simulink model "BMS_BalancingLogic_COM"  (R2022b)
settings: configuration reference "BMS_Sw_CodeGenConfig" (kept outside this file)
model workspace: external: MAT-File H:\0\New MAAM\10 - MBD\Battary Management System\SWE.3 CDD\DataTypes\Data_Script.mat (data not in the file)
undefined symbols (not defined in the file): Schedule
settings Model: DataDictionary=BMS_Arch_DD.sldd  Creator=MAAM  LastModifiedBy=MAAM
settings ConfigSetRef: SourceName=BMS_Sw_CodeGenConfig

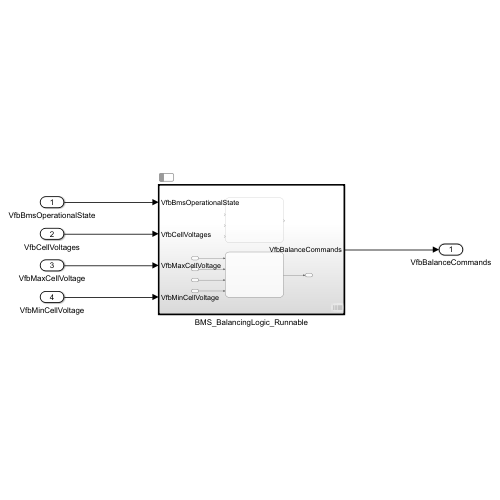
[thumbnail: Simulink's stored preview of the top-level diagram]
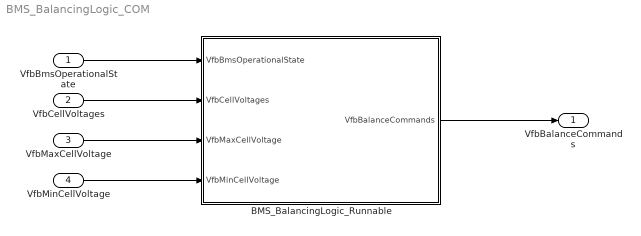
== system BMS_BalancingLogic_COM ==
  VfbBmsOperationalState : Inport
  VfbCellVoltages : Inport  Port=2
  VfbMaxCellVoltage : Inport  Port=3
  VfbMinCellVoltage : Inport  Port=4
  BMS_BalancingLogic_Runnable : Subsystem  Tag=BMS_BalancingLogic_Task  Priority=2  TreatAsAtomicUnit=on  ScheduleAs=Periodic partition  PartitionName=BMS_BalancingLogic_Task  SystemSampleTime=Schedule.BMS_BalancingLogic_Task
      settings: RTWSystemCode=Nonreusable function  RTWFcnNameOpts=Use subsystem name  RTWFileNameOpts=Use subsystem name  FunctionInterfaceSpec=Allow arguments (Optimized)
  VfbBalanceCommands : Outport
  wires:
  VfbBmsOperationalState/1 -> BMS_BalancingLogic_Runnable/1(VfbBmsOperationalState)
  VfbCellVoltages/1 -> BMS_BalancingLogic_Runnable/2(VfbCellVoltages)
  VfbMaxCellVoltage/1 -> BMS_BalancingLogic_Runnable/3(VfbMaxCellVoltage)
  VfbMinCellVoltage/1 -> BMS_BalancingLogic_Runnable/4(VfbMinCellVoltage)
  BMS_BalancingLogic_Runnable/1(VfbBalanceCommands) -> VfbBalanceCommands/1

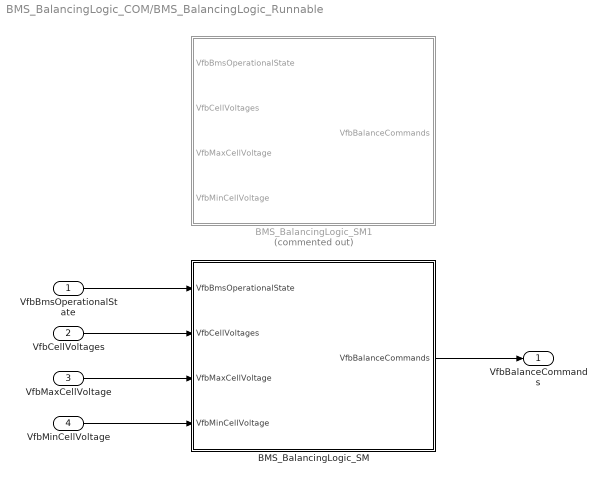
== system BMS_BalancingLogic_COM/BMS_BalancingLogic_Runnable ==
  VfbBmsOperationalState : Inport  OutDataTypeStr=Enum: BMS_State_Enum  PortDimensions=1
  VfbCellVoltages : Inport  Port=2
  VfbMaxCellVoltage : Inport  Port=3
  VfbMinCellVoltage : Inport  Port=4
  BMS_BalancingLogic_SM : Stateflow chart  TreatAsAtomicUnit=on
  BMS_BalancingLogic_SM1 : Stateflow chart  Commented=on  TreatAsAtomicUnit=on
  VfbBalanceCommands : Outport
  wires:
  VfbCellVoltages/1 -> BMS_BalancingLogic_SM/2(VfbCellVoltages)
  VfbMinCellVoltage/1 -> BMS_BalancingLogic_SM/4(VfbMinCellVoltage)
  BMS_BalancingLogic_SM/1(VfbBalanceCommands) -> VfbBalanceCommands/1
  VfbBmsOperationalState/1 -> BMS_BalancingLogic_SM/1(VfbBmsOperationalState)
  VfbMaxCellVoltage/1 -> BMS_BalancingLogic_SM/3(VfbMaxCellVoltage)

== stateflow chart BMS_BalancingLogic_COM/BMS_BalancingLogic_Runnable/BMS_BalancingLogic_SM ==
  state out  = ActivateBalancing(MAX, MIN, THR) [function]
    (default) -> (junction 25)
    (junction 25) -> (junction 26) [order 1] : [ (MAX - MIN) >= (THR - 1e-5) ]
    (junction 25) -> (junction 27) [order 2] : {out = false;}
    (junction 26) -> (junction 28) : {out = true;}
    (junction 28) -> (junction 27)
    (junction 27) -> (junction 29)
  state Balancing_Test [parallel]
    en, du:
    BalancingFlag = ActivateBalancing(VfbMaxCellVoltage, VfbMinCellVoltage, BalancingThreshold(state));
    settings: executionOrder=1
  state Balancing_Logic [parallel]
    settings: executionOrder=2
    state SW_Off
      en:
      VfbBalanceCommands(:,:) = false;
      state = 1;
    state Super
      state BalancingNotActive
        en:
        state = 1;
      state BalancingIsActive
        en, du:
        state = 2;
        VfbBalanceCommands(:,:) = boolean( (VfbCellVoltages - VfbMinCellVoltage)  > BalancingThreshold(state) );
        ex:
        VfbBalanceCommands(:,:) = false;
      (default) -> BalancingNotActive
      BalancingIsActive -> BalancingNotActive : [~BalancingFlag]
      BalancingNotActive -> BalancingIsActive [order 1] : [BalancingFlag]
    (default) -> SW_Off
    Super -> SW_Off : [VfbBmsOperationalState ~= BMS_State_Enum.BMS_Balancing]
    SW_Off -> Super : [BalancingFlag && ...
        | after(BalancingOffWait, sec)]
    BalancingNotActive -> SW_Off [order 2] : [after(BalancingOnWait, sec)]
  data: MAX function_input single size=1; out function_output boolean size=1; MIN function_input single size=1; THR function_input; VfbBmsOperationalState input Enum: BMS_State_Enum size=1; VfbCellVoltages input single size=BATT.Package.Ns_Module*BATT.Package.NumModules; VfbMaxCellVoltage input single size=1; VfbMinCellVoltage input single size=1; VfbBalanceCommands output boolean size=BATT.Package.Ns_Module*BATT.Package.NumModules =boolean(zeros(1,BATT.Package.Ns_Module*BATT.Package.NumModules))'; BalancingOffWait constant uint8 size=1 =BATT.Balancing.BalWaitOff; BalancingOnWait constant uint8 size=1 =BATT.Balancing.BalWaitOn; BalancingFlag local boolean size=1 =true; state local =1; BalancingThreshold constant single size=[1 2] =[BATT.Balancing.ThresholdOn , BATT.Balancing.ThresholdOff]

== stateflow chart BMS_BalancingLogic_COM/BMS_BalancingLogic_Runnable/BMS_BalancingLogic_SM1 ==
  state SW_Off
    en:
    VfbBalanceCommands(:,:) = false;
    du:
    BalancingFlag = ActivateBalancing(VfbMaxCellVoltage, VfbMinCellVoltage, BalancingThreshold_ON);
  state out  = ActivateBalancing(MAX, MIN, THR) [function]
    (default) -> (junction 25)
    (junction 25) -> (junction 26) [order 1] : [ (MAX - MIN) >= (THR - 1e-5) ]
    (junction 25) -> (junction 27) [order 2] : {out = false;}
    (junction 26) -> (junction 28) : {out = true;}
    (junction 28) -> (junction 27)
    (junction 27) -> (junction 29)
  state Super
    state BalancingNotActive
      en, du:
      BalancingFlag = ActivateBalancing(VfbMaxCellVoltage, VfbMinCellVoltage, BalancingThreshold_ON);
    state BalancingIsActive
      en, du:
      BalancingFlag = ActivateBalancing( ...
      VfbMaxCellVoltage, VfbMinCellVoltage, BalancingThreshold_OFF);
      ex:
      VfbBalanceCommands(:,:) = false;
      state BalancingActiveMode
        state SW1_On
          en:
          VfbBalanceCommands(1) = true;
          ex:
          VfbBalanceCommands(1) = false;
          step = 1;
        state SW_Wait
        state SW2_On
          en:
          VfbBalanceCommands(2) = true;
          ex:
          VfbBalanceCommands(2) = false;
          step = 2;
        (default) -> SW1_On
        SW_Wait -> SW1_On [order 1] : after((0.5-Don)/Freq, sec)[step >= 2]
        SW1_On -> SW_Wait : after(Don/Freq - 0.0001, sec)
        SW_Wait -> SW2_On [order 2] : after((0.5-Don)/Freq, sec)[step <= 1]
        SW2_On -> SW_Wait : after(Don/Freq - 0.0001, sec)
      state BalancingPassiveMode
        en, du:
        VfbBalanceCommands(:,:) = boolean( ...
        (VfbCellVoltages - VfbMinCellVoltage) > BalancingThreshold_OFF);
      (default) -> (junction 113)
      (junction 113) -> BalancingActiveMode [order 1] : [BalancingMode]
      (junction 113) -> BalancingPassiveMode [order 2]
    (default) -> BalancingNotActive
    BalancingIsActive -> BalancingNotActive : [~BalancingFlag]
    BalancingNotActive -> BalancingIsActive [order 1] : [BalancingFlag]
  (default) -> SW_Off
  Super -> SW_Off : [VfbBmsOperationalState == BMS_State_Enum.BMS_Driving || ...
      | VfbBmsOperationalState == BMS_State_Enum.BMS_Fault]
  SW_Off -> Super : [BalancingFlag && ...
      | after(BalancingOffWait, sec)]
  BalancingNotActive -> SW_Off [order 2] : [after(BalancingOnWait, sec)]
  data: MAX function_input single size=1; out function_output boolean size=1; MIN function_input single size=1; THR function_input; VfbBmsOperationalState input Enum: BMS_State_Enum size=1; VfbCellVoltages input single size=BATT.Package.Ns_Module*BATT.Package.NumModules; VfbMaxCellVoltage input single size=1; VfbMinCellVoltage input single size=1; VfbBalanceCommands output boolean size=BATT.Package.Ns_Module*BATT.Package.NumModules =boolean(zeros(1,BATT.Package.Ns_Module*BATT.Package.NumModules))'; Don constant single size=1 =BATT.Balancing.Duty; Freq constant single size=1 =BATT.Balancing.Freq; BalancingThreshold_ON constant single size=1 =BATT.Balancing.ThresholdOn; step local single size=1 =single(1); BalancingOffWait constant uint8 size=1 =BATT.Balancing.BalWaitOff; BalancingOnWait constant uint8 size=1 =BATT.Balancing.BalWaitOn; BalancingFlag local boolean size=1 =true; BalancingMode constant boolean size=1 =BATT.Balancing.Mode; BalancingThreshold_OFF constant single size=1 =BATT.Balancing.ThresholdOff
